simulink library "TireBody_Models"  (R2023a)
settings: Solver=VariableStepAuto  StartTime=0.0  StopTime=10.0  RelTol=1e-3
undefined symbols (not defined in the file): tyre_Ixx, tyre_Iyy, Vehicle
libraries: Bus_Makhulu_Parts x2, Truck_Amandla_Parts x2, Trailer_Thwala_Parts x1, Sedan_Hamba_Parts x1, sm_lib x1, TireBody_Parameterized x1
Description:
  | Component of Simscape Vehicle Templates Library
  | 
  | Copyright 2018-2023 The MathWorks, Inc.
settings Model: Creator=smiller  LastModifiedBy=smiller
settings SolverCC: AlgebraicLoopSolver=TrustRegion
settings DataIOCC: ReturnWorkspaceOutputs=off
settings OptimizationCC: ReuseModelBlockBuffer=off
settings DebuggingCC: UnconnectedInputMsg=warning  UnconnectedOutputMsg=warning  UnconnectedLineMsg=warning  ArithmeticOperatorsInVariantConditions=warning
settings ModelReferenceCC: EnableRefExpFcnMdlSchedulingChecks=on
settings SFSimCC: CustomCodeUndefinedFunction=UseInterfaceOnly

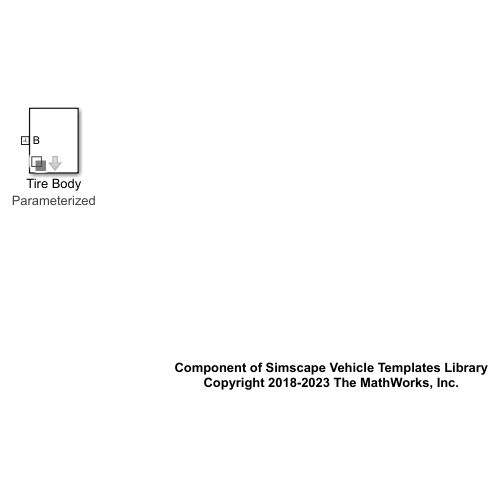
[thumbnail: Simulink's stored preview of the top-level diagram]
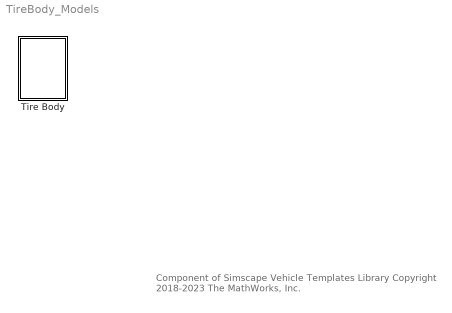
== system TireBody_Models ==
  note: Component of Simscape Vehicle Templates Library
      | Copyright 2018-2023 The MathWorks, Inc.
  Tire Body : Subsystem  Variant=on  VariantControlMode=label  LabelModeActiveChoice=Parameterized  mask(Variants for Tire Body){popup_leftRight=Right, TireBody=Vehicle.Chassis.TireA1.TireBody, VariantLabel=Vehicle.Chassis.TireA1.TireBody.class.Value, InitTriggerDropdown=1}
      mask prompts: popup_leftRight "Left/Right"; TireBody "Tire Body (structure)"; VariantLabel "Variant Label"; InitTriggerDropdown "Initialization Dropdown Trigger"
      mask help: Select option and provide parameters for tire geometry, mass, and inertia. Option is chosen by string provided in Variant Label. The parameters for the selected option is contained in TireBody data structure.
      mask init:
      | curblk = gcb;
      | 
      | tirbody_variant = get_param(gcb,'ActiveVariant');
      | if (popup_leftRight == 1)
      |     if(strcmp(tirbody_variant,'Parameterized'))
      |         set_param([gcb '/Parameterized'],'popup_leftRight','Left');
      |     elseif(strcmp(tirbody_variant,'CAD_145_70R13'))
      |         set_param([gcb '/CAD_145_70R13'],'popup_leftRight','Left');
      |     elseif(strcmp(tirbody_variant,'CAD_213_40R21'))
      |         set_param([gcb '/CAD_213_40R21'],'popup_leftRight','Left');
      |     elseif(strcmp(tirbody_variant,'CAD_270_70R22'))
      |         set_param([gcb '/CAD_270_70R22'],'popup_leftRight','Left');
      |     elseif(strcmp(tirbody_variant,'CAD_270_70R22_2x'))
      |         set_param([gcb '/CAD_270_70R22_2x'],'popup_leftRight','Left');
      |     elseif(strcmp(tirbody_variant,'CAD_430_50R38'))
      |         set_param([gcb '/CAD_430_50R38'],'popup_leftRight','Left');
      |     elseif(strcmp(tirbody_variant,'CAD_430_50R38_2x'))
      |         set_param([gcb '/CAD_430_50R38_2x'],'popup_leftRight','Left');
      |     end
      | elseif (popup_leftRight == 2)
      |     if(strcmp(tirbody_variant,'Parameterized'))
      |         set_param([gcb '/Parameterized'],'popup_leftRight','Right');
      |     elseif(strcmp(tirbody_variant,'CAD_145_70R13'))
      |         set_param([gcb '/CAD_145_70R13'],'popup_leftRight','Right');
      |     elseif(strcmp(tirbody_variant,'CAD_213_40R21'))
      |         set_param([gcb '/CAD_213_40R21'],'popup_leftRight','Right');
      |     elseif(strcmp(tirbody_variant,'CAD_270_70R22'))
      |         set_param([gcb '/CAD_270_70R22'],'popup_leftRight','Right');
      |     elseif(strcmp(tirbody_variant,'CAD_270_70R22_2x'))
      |         set_param([gcb '/CAD_270_70R22_2x'],'popup_leftRight','Right');
      |     elseif(strcmp(tirbody_variant,'CAD_430_50R38'))
      |         set_param([gcb '/CAD_430_50R38'],'popup_leftRight','Right');
      |     elseif(strcmp(tirbody_variant,'CAD_430_50R38_2x'))
      |         set_param([gcb '/CAD_430_50R38_2x'],'popup_leftRight','Right');
      |     end
      | end
      | 
      | 
      | % Set variant for this block 
      | set_param(curblk,'LabelModeActiveChoice',VariantLabel);
      | 
      | % Trigger Mask Initialization for 
      | % variant subsystems below this level
      | sm_car_lib_maskInitTrigger(curblk);
      settings: AttributesFormatString=%<LabelModeActiveChoice>
      mask TypeOptions popup_leftRight: Left | Right
      mask TypeOptions InitTriggerDropdown: 0 | 1
      mask Display: disp(' ');

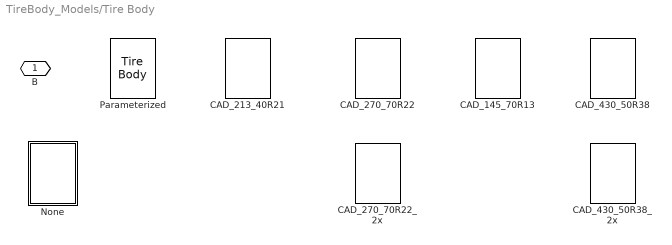
== system TireBody_Models/Tire Body ==
  CAD_145_70R13 : Trailer_Thwala_Parts/CAD_145_70R13  VariantControl=CAD_145_70R13  LabelModeActiveChoice=Left  popup_leftRight=Left  mass_tire=tyre_mass  mass_rim=0  tire_inertia=[tyre_Ixx tyre_Iyy]  rim_inertia=[0 0]  offset_cg=[0 0 0]
      settings: AttributesFormatString=%<LabelModeActiveChoice>
  CAD_213_40R21 : Sedan_Hamba_Parts/CAD_213_40R21  VariantControl=CAD_213_40R21  LabelModeActiveChoice=Right  popup_leftRight=Right  mass_tire=tyre_mass  mass_rim=0  tire_inertia=[tyre_Ixx tyre_Iyy]  rim_inertia=[0 0]  offset_cg=[0 0 0]
      settings: AttributesFormatString=%<LabelModeActiveChoice>
  CAD_270_70R22 : Bus_Makhulu_Parts/CAD_270_70R22  VariantControl=CAD_270_70R22  LabelModeActiveChoice=Right  popup_leftRight=Right  mass_tire=tyre_mass  mass_rim=0  tire_inertia=[tyre_Ixx tyre_Iyy]  rim_inertia=[0 0]  offset_cg=[0 0 0]  InitDropdownTrigger=0
      settings: AttributesFormatString=%<LabelModeActiveChoice>
  CAD_270_70R22_2x : Bus_Makhulu_Parts/CAD_270_70R22_2x  VariantControl=CAD_270_70R22_2x  LabelModeActiveChoice=Left  popup_leftRight=Left  mass_tire=tyre_mass  mass_rim=0  tire_inertia=[tyre_Ixx tyre_Iyy]  rim_inertia=[0 0]  offset_cg=[0 0 0]  InitDropdownTrigger=0
      settings: AttributesFormatString=%<LabelModeActiveChoice>
  CAD_430_50R38 : Truck_Amandla_Parts/CAD_430_50R38  VariantControl=CAD_430_50R38  LabelModeActiveChoice=Left  popup_leftRight=Left  mass_tire=tyre_mass  mass_rim=0  tire_inertia=[tyre_Ixx tyre_Iyy]  rim_inertia=[0 0]  offset_cg=[0 0 0]  InitDropdownTrigger=0
      settings: AttributesFormatString=%<LabelModeActiveChoice>
  CAD_430_50R38_2x : Truck_Amandla_Parts/CAD_430_50R38_2x  VariantControl=CAD_430_50R38_2x  LabelModeActiveChoice=Left  popup_leftRight=Left  mass_tire=tyre_mass  mass_rim=0  tire_inertia=[tyre_Ixx tyre_Iyy]  rim_inertia=[0 0]  offset_cg=[0 0 0]  InitDropdownTrigger=0
      settings: AttributesFormatString=%<LabelModeActiveChoice>
  None : Subsystem  VariantControl=None
  Parameterized : TireBody_Parameterized/Tire Body  VariantControl=Parameterized  radius=tire_radius  rim_radius=rim_radius  width=tire_width  rim_width=rim_width  mass=tyre_mass  rim_mass=0  tire_inertia=[tyre_Ixx tyre_Iyy]  rim_inertia=[0 0]  popup_leftRight=Left  clr_tyre=Visual.Tire.clr  opc_tyre=Visual.Tire.opc  clr_rim=Visual.Rim.clr  opc_rim=Visual.Rim.opc
  B : PMIOPort  Side=Left

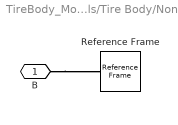
== system TireBody_Models/Tire Body/None ==
  Reference Frame : sm_lib/Frames and Transforms/Reference Frame
  B : PMIOPort  Side=Left
  connections:
  B/RConn1 -- Reference Frame/RConn1
